simulink model "ozgur"  (R2016a)
settings: Solver=ode4  SolverMode=SingleTasking  StartTime=0.0  StopTime=0.08  FixedStep=1e-5  RelTol=1e-3
libraries: powerlib_meascontrol x14, arduino_io_lib x4
settings Model: ExtModeTrigDuration=2  Creator=gcampa  LastModifiedBy=syf
settings DataIOCC: LimitDataPoints=on  SaveFormat=Array  SignalLoggingSaveFormat=ModelDataLogs
settings OptimizationCC: OptimizeModelRefInitCode=on  LifeSpan=1  MaxStackSize=64
settings DebuggingCC: UnderspecifiedInitializationDetection=Classic  MergeDetectMultiDrivingBlocksExec=none  MultiTaskDSMMsg=warning  MultiTaskCondExecSysMsg=none
settings HardwareCC: ProdBitPerInt=16  ProdBitPerPointer=16  ProdLargestAtomicFloat=None  ProdWordSize=8  ProdHWDeviceType=Atmel->AVR
settings ModelReferenceCC: PropagateSignalLabelsOutOfModel=off
settings RTWCC: SystemTargetFile=ert.tlc  HardwareBoard=Arduino Uno  TemplateMakefile=ert_default_tmf  GenerateReport=on  RTWVerbose=off  Toolchain=Arduino AVR v1.6.1  BuildConfiguration=Faster Runs  IncludeHyperlinkInReport=on  LaunchReport=on  GenerateTraceInfo=on  GenerateTraceReport=on  GenerateTraceReportSl=on  GenerateTraceReportSf=on  GenerateTraceReportEml=on
settings CodeAppCC: ForceParamTrailComments=on  IgnoreCustomStorageClasses=off  OperatorAnnotations=on  SimulinkDataObjDesc=on  SFDataObjDesc=on  MATLABFcnDesc=on  InsertBlockDesc=on  MATLABSourceComments=on
settings ERTTargetCC: SupportContinuousTime=on  SupportVariableSizeSignals=on
settings ConfigComp: CovModelRefEnable=Off

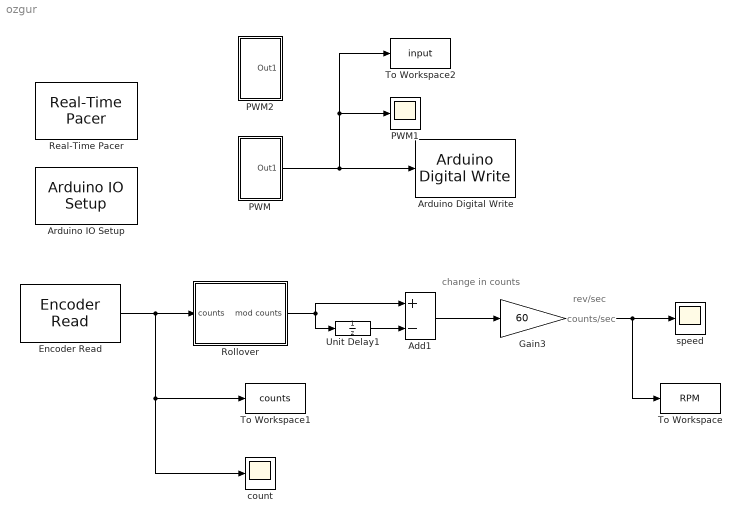
== system ozgur ==
  note: change
      | in counts
  note: rev/sec
  note: counts/sec
  Add1 : Sum  Inputs=+-
  Arduino Digital Write : arduino_io_lib/Arduino Digital Write  arduinoVar=Temporary arduino variable: Arduino1  arduinoPin=6  T=1e-5
  Arduino IO Setup : arduino_io_lib/Arduino IO Setup  Priority=3  arduinoVar=Temporary arduino variable: Arduino1  workspaceVarName=a  comPort=COM5
  Encoder Read : arduino_io_lib/Encoder Read  arduinoVar=Temporary arduino variable: Arduino1  encNum=1  pinA=3  pinB=2  DbDl=0  T=1e-5
  Gain3 : Gain  Gain=60
  PWM : Subsystem
  PWM1 : Scope
  PWM2 : Subsystem
  Real-Time Pacer : arduino_io_lib/Real-Time Pacer  simTimePerRealTime=1
  Rollover : Subsystem
  To Workspace : ToWorkspace  VariableName=RPM  SampleTime=-1
  To Workspace1 : ToWorkspace  VariableName=counts  SampleTime=-1
  To Workspace2 : ToWorkspace  VariableName=input  SampleTime=-1
  Unit Delay1 : UnitDelay  SampleTime=1e-5
  count : Scope
  speed : Scope
  wires:
  Unit Delay1/1 -> Add1/2
  Rollover/1(" mod counts") -> Add1/1, Unit Delay1/1
  Encoder Read/1 -> Rollover/1(counts), count/1, To Workspace1/1
  Gain3/1 -> speed/1, To Workspace/1
  PWM/1(Out1) -> To Workspace2/1, PWM1/1, Arduino Digital Write/1
  Add1/1 -> Gain3/1

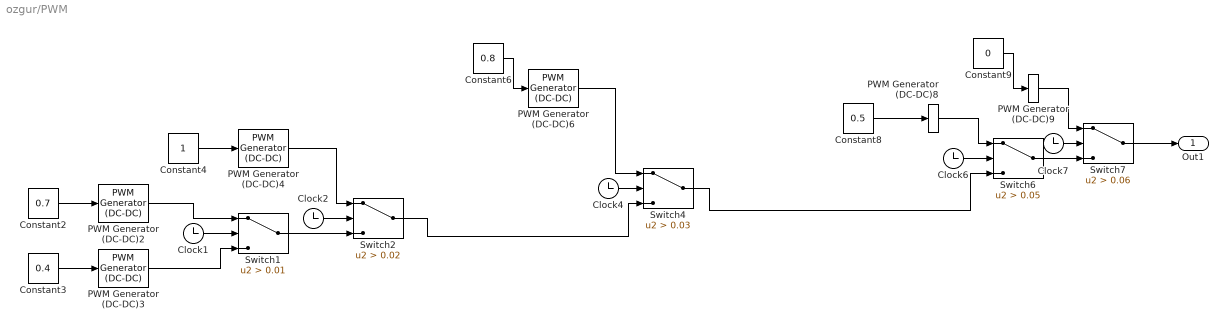
== system ozgur/PWM ==
  Clock{1..2,4,6..7} (5 alike) : Clock
  Constant2 : Constant  Value=0.7
  Constant3 : Constant  Value=0.4
  Constant4 : Constant
  Constant6 : Constant  Value=0.8
  Constant8 : Constant  Value=0.5
  Constant9 : Constant  Value=0
  PWM Generator (DC-DC){2..4,6,8..9} (6 alike) : powerlib_meascontrol/Pulse & Signal Generators/PWM Generator (DC-DC)  Fsw=5000  Ts=1e-5
  Switch1 : Switch  Criteria=u2 > Threshold  Threshold=0.01
  Switch2 : Switch  Criteria=u2 > Threshold  Threshold=0.02
  Switch4 : Switch  Criteria=u2 > Threshold  Threshold=0.03
  Switch6 : Switch  Criteria=u2 > Threshold  Threshold=0.05
  Switch7 : Switch  Criteria=u2 > Threshold  Threshold=0.06
  Out1 : Outport
  wires:
  Clock6/1 -> Switch6/2
  Clock4/1 -> Switch4/2
  Clock7/1 -> Switch7/2
  Constant4/1 -> PWM Generator (DC-DC)4/1
  PWM Generator (DC-DC)4/1 -> Switch2/1
  PWM Generator (DC-DC)6/1 -> Switch4/1
  Constant6/1 -> PWM Generator (DC-DC)6/1
  Switch4/1 -> Switch6/3
  PWM Generator (DC-DC)2/1 -> Switch1/1
  Clock1/1 -> Switch1/2
  PWM Generator (DC-DC)3/1 -> Switch1/3
  Constant3/1 -> PWM Generator (DC-DC)3/1
  Constant2/1 -> PWM Generator (DC-DC)2/1
  PWM Generator (DC-DC)9/1 -> Switch7/1
  Switch1/1 -> Switch2/3
  Switch2/1 -> Switch4/3
  Clock2/1 -> Switch2/2
  Switch6/1 -> Switch7/3
  Constant9/1 -> PWM Generator (DC-DC)9/1
  Switch7/1 -> Out1/1
  Constant8/1 -> PWM Generator (DC-DC)8/1
  PWM Generator (DC-DC)8/1 -> Switch6/1

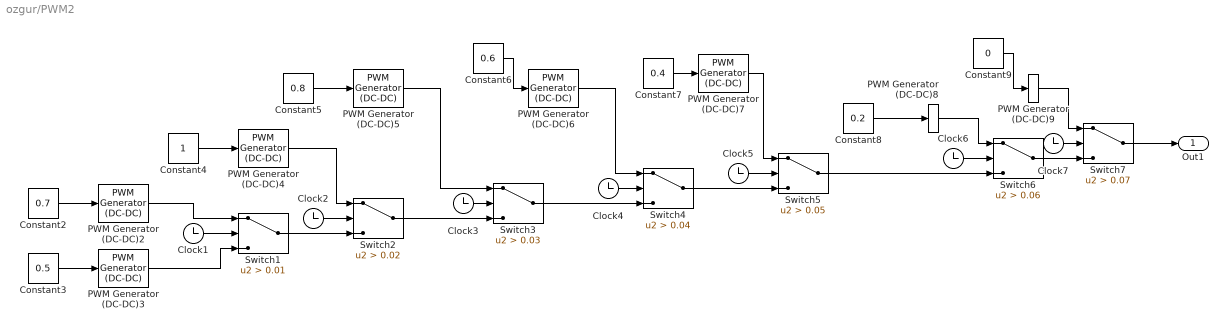
== system ozgur/PWM2 ==
  Clock{1..7} (7 alike) : Clock
  Constant2 : Constant  Value=0.7
  Constant3 : Constant  Value=0.5
  Constant4 : Constant
  Constant5 : Constant  Value=0.8
  Constant6 : Constant  Value=0.6
  Constant7 : Constant  Value=0.4
  Constant8 : Constant  Value=0.2
  Constant9 : Constant  Value=0
  PWM Generator (DC-DC){2..9} (8 alike) : powerlib_meascontrol/Pulse & Signal Generators/PWM Generator (DC-DC)  Fsw=5000  Ts=1e-5
  Switch1 : Switch  Criteria=u2 > Threshold  Threshold=0.01
  Switch2 : Switch  Criteria=u2 > Threshold  Threshold=0.02
  Switch3 : Switch  Criteria=u2 > Threshold  Threshold=0.03
  Switch4 : Switch  Criteria=u2 > Threshold  Threshold=0.04
  Switch5 : Switch  Criteria=u2 > Threshold  Threshold=0.05
  Switch6 : Switch  Criteria=u2 > Threshold  Threshold=0.06
  Switch7 : Switch  Criteria=u2 > Threshold  Threshold=0.07
  Out1 : Outport
  wires:
  Switch4/1 -> Switch5/3
  PWM Generator (DC-DC)8/1 -> Switch6/1
  Constant8/1 -> PWM Generator (DC-DC)8/1
  Switch7/1 -> Out1/1
  Constant9/1 -> PWM Generator (DC-DC)9/1
  Switch6/1 -> Switch7/3
  Clock2/1 -> Switch2/2
  Constant5/1 -> PWM Generator (DC-DC)5/1
  Switch2/1 -> Switch3/3
  PWM Generator (DC-DC)5/1 -> Switch3/1
  Constant7/1 -> PWM Generator (DC-DC)7/1
  PWM Generator (DC-DC)7/1 -> Switch5/1
  Switch3/1 -> Switch4/3
  Switch1/1 -> Switch2/3
  PWM Generator (DC-DC)9/1 -> Switch7/1
  Constant2/1 -> PWM Generator (DC-DC)2/1
  Constant3/1 -> PWM Generator (DC-DC)3/1
  PWM Generator (DC-DC)3/1 -> Switch1/3
  Clock1/1 -> Switch1/2
  PWM Generator (DC-DC)2/1 -> Switch1/1
  Switch5/1 -> Switch6/3
  Constant6/1 -> PWM Generator (DC-DC)6/1
  PWM Generator (DC-DC)6/1 -> Switch4/1
  PWM Generator (DC-DC)4/1 -> Switch2/1
  Constant4/1 -> PWM Generator (DC-DC)4/1
  Clock7/1 -> Switch7/2
  Clock4/1 -> Switch4/2
  Clock3/1 -> Switch3/2
  Clock6/1 -> Switch6/2
  Clock5/1 -> Switch5/2

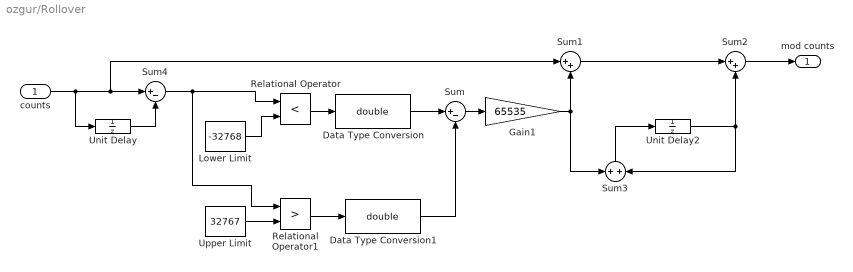
== system ozgur/Rollover ==
  counts : Inport
  " Lower Limit" : Constant  Value=-32768
  " Upper Limit" : Constant  Value=32767
  Data Type Conversion : DataTypeConversion  OutDataTypeStr=double  RndMeth=Zero
  Data Type Conversion1 : DataTypeConversion  OutDataTypeStr=double  RndMeth=Zero
  Gain1 : Gain  Gain=65535
  Relational Operator : RelationalOperator  Operator=<  OutDataTypeStr=boolean
  Relational Operator1 : RelationalOperator  Operator=>  OutDataTypeStr=boolean
  Sum : Sum  Inputs=|+-
  Sum1 : Sum  Inputs=|++
  Sum2 : Sum  Inputs=|++
  Sum3 : Sum
  Sum4 : Sum  Inputs=|+-
  Unit Delay : UnitDelay  SampleTime=-1
  Unit Delay2 : UnitDelay  SampleTime=-1
  " mod counts" : Outport
  wires:
  counts/1 -> Unit Delay/1, Sum1/1, Sum4/1
  Sum2/1 -> " mod counts"/1
  Unit Delay/1 -> Sum4/2
  Data Type Conversion/1 -> Sum/1
  Sum3/1 -> Unit Delay2/1
  Data Type Conversion1/1 -> Sum/2
  Sum/1 -> Gain1/1
  Gain1/1 -> Sum1/2, Sum3/1
  Relational Operator1/1 -> Data Type Conversion1/1
  Sum1/1 -> Sum2/1
  Relational Operator/1 -> Data Type Conversion/1
  " Upper Limit"/1 -> Relational Operator1/2
  Unit Delay2/1 -> Sum3/2, Sum2/2
  " Lower Limit"/1 -> Relational Operator/2
  Sum4/1 -> Relational Operator/1, Relational Operator1/1
